simulink model "BAllowTorque"  (R2024b)
settings: configuration reference "STM32H7_Config" (kept outside this file)
undefined symbols (not defined in the file): IMaxAllowed, nMotorMax
libraries: simulink x2
settings Model: DataDictionary=Master_Dictionary.sldd  EnableAccessToBaseWorkspace=off  Creator=torni  LastModifiedBy=Will
settings ConfigSetRef: SourceName=STM32H7_Config

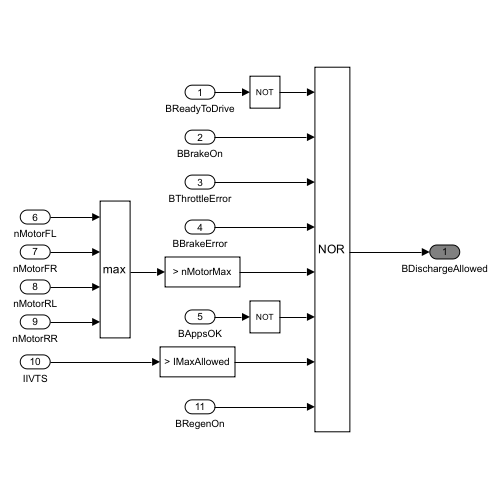
[thumbnail: Simulink's stored preview of the top-level diagram]
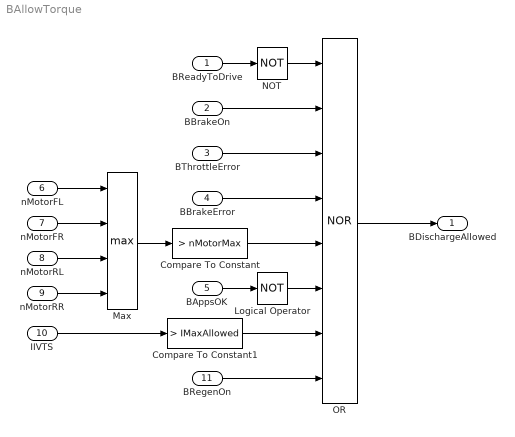
== system BAllowTorque ==
  "BReadyToDrive " : Inport  OutDataTypeStr=boolean
  BBrakeOn : Inport  Port=2  OutDataTypeStr=boolean
  BThrottleError : Inport  Port=3  OutDataTypeStr=boolean
  BBrakeError : Inport  Port=4  OutDataTypeStr=boolean
  BAppsOK : Inport  Port=5  OutDataTypeStr=boolean
  nMotorFL : Inport  Port=6  OutDataTypeStr=double
  nMotorFR : Inport  Port=7  OutDataTypeStr=double
  nMotorRL : Inport  Port=8  OutDataTypeStr=double
  nMotorRR : Inport  Port=9  OutDataTypeStr=double
  IIVTS : Inport  Port=10  OutDataTypeStr=double
  BRegenOn : Inport  Port=11  OutDataTypeStr=boolean
  Compare To Constant : simulink/Logic and Bit Operations/Compare To Constant  relop=>  const=nMotorMax  OutDataTypeStr=boolean
  Compare To Constant1 : simulink/Logic and Bit Operations/Compare To Constant  relop=>  const=IMaxAllowed  OutDataTypeStr=boolean
  Logical Operator : Logic  Operator=NOT  AllPortsSameDT=off  OutDataTypeStr=boolean
  Max : MinMax  Function=max  Inputs=4
  NOT : Logic  Operator=NOT  AllPortsSameDT=off  OutDataTypeStr=boolean
  OR : Logic  Operator=NOR  Inputs=8  AllPortsSameDT=off  OutDataTypeStr=boolean
  BDischargeAllowed : Outport  OutDataTypeStr=boolean  VectorParamsAs1DForOutWhenUnconnected=off
  wires:
  "BReadyToDrive "/1 -> NOT/1
  BBrakeOn/1 -> OR/2
  BThrottleError/1 -> OR/3
  BAppsOK/1 -> Logical Operator/1
  Logical Operator/1 -> OR/6
  Max/1 -> Compare To Constant/1
  Compare To Constant/1 -> OR/5
  nMotorRR/1 -> Max/4
  nMotorRL/1 -> Max/3
  nMotorFR/1 -> Max/2
  nMotorFL/1 -> Max/1
  NOT/1 -> OR/1
  OR/1 -> BDischargeAllowed/1
  IIVTS/1 -> Compare To Constant1/1
  Compare To Constant1/1 -> OR/7
  BBrakeError/1 -> OR/4
  BRegenOn/1 -> OR/8
